simulink model "H8_EMS_partelinealizada"  (R2022b)
settings: Solver=VariableStepAuto  StartTime=0.0  StopTime=10.0  RelTol=1e-3
InitFcn:
  | m = 200;
  | g = 9.81;
  | x_lev12 = 0.443;
  | x_lev34 = 0.542;
  | x_guid12 = 0.4475;
  | x_guid34 = 0.5465;
  | x_lim = 0.0495;
  | y_lev13 = 0.23686;
  | y_lev24 = 0.23686;
  | y_guid13 = 0.24263;
  | y_guid24 = 0.24263;
  | y_lim = 0.0005;
  | y_brk = 0.21552;
  | z_lev = 0.08546;
  | z_guid = 0.026;
  | z_lim = 0.1055;
  | z_brk = 0.03941;
  | kp_lev = 50;
  | ki_lev = 400;
  | kp_guid = 6;
  | ki_guid = 46.5;
  | Imax_lev = 50;
  | Imin_lev = -50;
  | Imax_guid = 50;
  | Imin_guid = 0;
  | cg_nom = 0.567;
  | I = [43.082 0 0; 0 26.887 0; 0 0 29.297]
values from neighbouring files (symbols this model uses):
  cg_suelo = 0.56985    [linealizacion_HEMS.m]
  cg_techo = 0.55735    [linealizacion_HEMS.m]
undefined symbols (not defined in the file or in its folder): ems
libraries: shared6dof x1
settings Model: Creator=USUARIO  LastModifiedBy=USUARIO

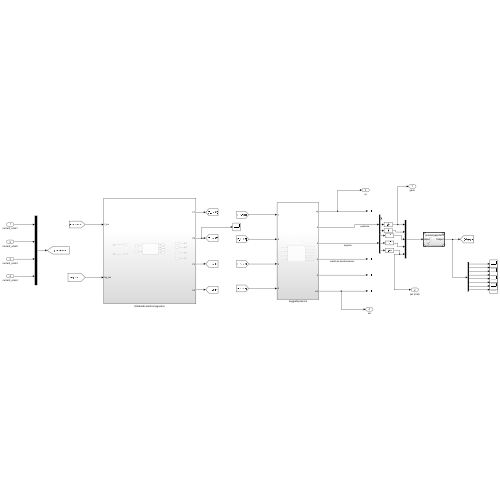
[thumbnail: Simulink's stored preview of the top-level diagram]
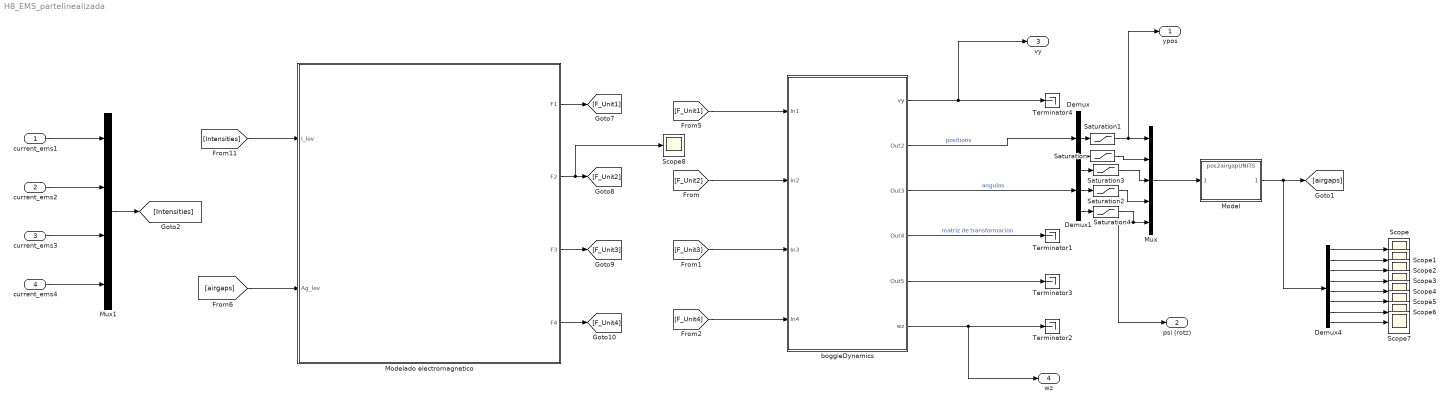
== system H8_EMS_partelinealizada ==
  current_ems1 : Inport
  current_ems2 : Inport  Port=2
  current_ems3 : Inport  Port=3
  current_ems4 : Inport  Port=4
  Demux : Demux  Outputs=3
  Demux1 : Demux  Outputs=3
  Demux4 : Demux  Outputs=8
  Model : ModelReference  ModelNameDialog=pos2airgapUNITS.slx  SimulationMode=Normal  ModelReferenceVersion=1.3
  Modelado electromagnetico : Subsystem
  Mux : Mux  Inputs=5
  Mux1 : Mux
  Saturation : Saturate  UpperLimit=cg_suelo  LowerLimit=cg_techo
  Saturation1 : Saturate  UpperLimit=0.012  LowerLimit=-0.012
  Saturation2 : Saturate  UpperLimit=0.01268  LowerLimit=-0.01268
  Saturation3 : Saturate  UpperLimit=0.0476  LowerLimit=-0.0476
  Saturation4 : Saturate  UpperLimit=0.024  LowerLimit=-0.024
  Scope{,1..8} (9 alike) : Scope
  Terminator{1..4} (4 alike) : Terminator
  boggieDynamics : Subsystem
  ypos : Outport
  psi (rotz) : Outport  Port=2
  vy : Outport  Port=3
  wz : Outport  Port=4
  wires:
  boggieDynamics/3(Out3) -> Demux1/1  "angulos"
  Saturation1/1 -> Mux/1, ypos/1
  boggieDynamics/6(wz) -> wz/1, Terminator2/1
  current_ems3/1 -> Mux1/3
  Demux1/2 -> Saturation2/1
  Demux4/1 -> Scope/1
  boggieDynamics/4(Out4) -> Terminator1/1  "matriz de transformacion"
  Demux4/7 -> Scope6/1
  Saturation/1 -> Mux/2
  current_ems1/1 -> Mux1/1
  [Intensities] -> Modelado electromagnetico/1(I_lev)
  Demux/3 -> Saturation/1
  Demux/2 -> Saturation1/1
  Demux4/4 -> Scope3/1
  Model/1 -> Demux4/1, [airgaps]
  Demux4/3 -> Scope2/1
  Demux4/6 -> Scope5/1
  Saturation4/1 -> psi (rotz)/1, Mux/5
  Mux/1 -> Model/1
  Saturation2/1 -> Mux/4
  Modelado electromagnetico/1(F1) -> [F_Unit1]
  Demux4/8 -> Scope7/1
  [airgaps] -> Modelado electromagnetico/2(Ag_lev)
  Modelado electromagnetico/4(F4) -> [F_Unit4]
  Demux4/2 -> Scope1/1
  Demux4/5 -> Scope4/1
  Demux1/1 -> Saturation3/1
  Demux1/3 -> Saturation4/1
  Saturation3/1 -> Mux/3
  Modelado electromagnetico/3(F3) -> [F_Unit3]
  current_ems4/1 -> Mux1/4
  boggieDynamics/2(Out2) -> Demux/1  "positions"
  Mux1/1 -> [Intensities]
  boggieDynamics/5(Out5) -> Terminator3/1
  boggieDynamics/1(vy) -> vy/1, Terminator4/1
  current_ems2/1 -> Mux1/2
  Modelado electromagnetico/2(F2) -> Scope8/1, [F_Unit2]
  [F_Unit1] -> boggieDynamics/1(In1)
  [F_Unit4] -> boggieDynamics/4(In4)
  [F_Unit3] -> boggieDynamics/3(In3)
  [F_Unit2] -> boggieDynamics/2(In2)

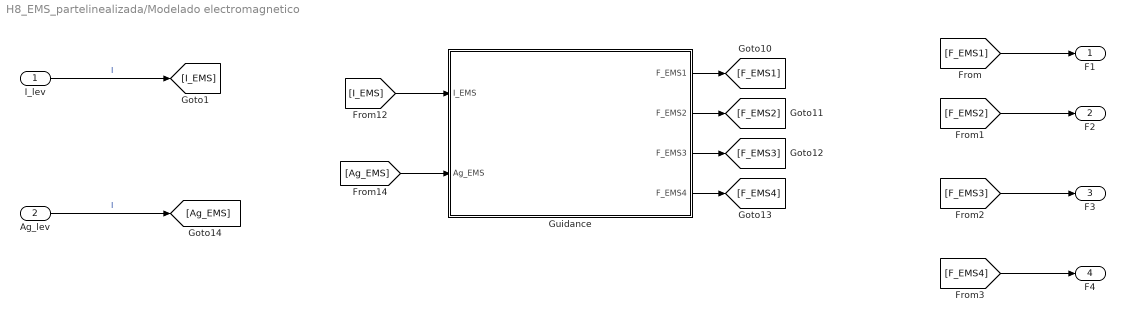
== system H8_EMS_partelinealizada/Modelado electromagnetico ==
  I_lev : Inport
  Ag_lev : Inport  Port=2
  Guidance : Subsystem
  F1 : Outport
  F2 : Outport  Port=2
  F3 : Outport  Port=3
  F4 : Outport  Port=4
  wires:
  I_lev/1 -> [I_EMS]  "I"
  Guidance/2(F_EMS2) -> [F_EMS2]
  Guidance/3(F_EMS3) -> [F_EMS3]
  Guidance/4(F_EMS4) -> [F_EMS4]
  Guidance/1(F_EMS1) -> [F_EMS1]
  [I_EMS] -> Guidance/1(I_EMS)
  [Ag_EMS] -> Guidance/2(Ag_EMS)
  Ag_lev/1 -> [Ag_EMS]  "I"
  [F_EMS2] -> F2/1
  [F_EMS1] -> F1/1
  [F_EMS3] -> F3/1
  [F_EMS4] -> F4/1

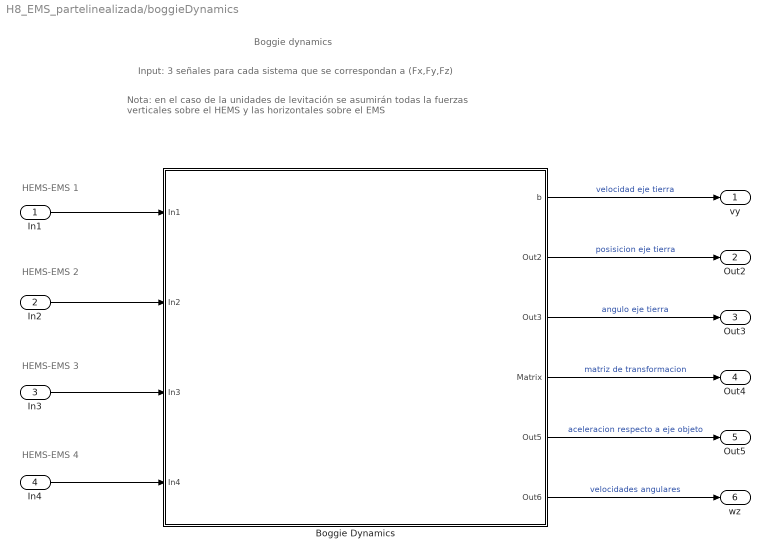
== system H8_EMS_partelinealizada/boggieDynamics ==
  note: Input: 3 señales para cada sistema que se correspondan a (Fx,Fy,Fz)
  note: HEMS-EMS 3
  note: HEMS-EMS 1
  note: HEMS-EMS 4
  note: HEMS-EMS 2
  note: Boggie dynamics
  note: Nota: en el caso de la unidades de levitación se asumirán todas la fuerzas
      | verticales sobre el HEMS y las horizontales sobre el EMS
  In1 : Inport
  In2 : Inport  Port=2
  In3 : Inport  Port=3
  In4 : Inport  Port=4
  Boggie Dynamics : Subsystem
      mask Display: image('C:\UPV\Hyperloop\Levitacion\ejes.png'); % Use "Edit Image" on toolstrip to change.
  vy : Outport
  Out2 : Outport  Port=2
  Out3 : Outport  Port=3
  Out4 : Outport  Port=4
  Out5 : Outport  Port=5
  wz : Outport  Port=6
  wires:
  Boggie Dynamics/4(Matrix) -> Out4/1  "matriz de transformacion"
  Boggie Dynamics/6(Out6) -> wz/1  "velocidades angulares"
  Boggie Dynamics/5(Out5) -> Out5/1  "aceleracion respecto a eje objeto"
  In1/1 -> Boggie Dynamics/1(In1)
  In3/1 -> Boggie Dynamics/3(In3)
  In4/1 -> Boggie Dynamics/4(In4)
  Boggie Dynamics/1(b) -> vy/1  "velocidad eje tierra"
  In2/1 -> Boggie Dynamics/2(In2)
  Boggie Dynamics/2(Out2) -> Out2/1  "posisicion eje tierra"
  Boggie Dynamics/3(Out3) -> Out3/1  "angulo eje tierra"

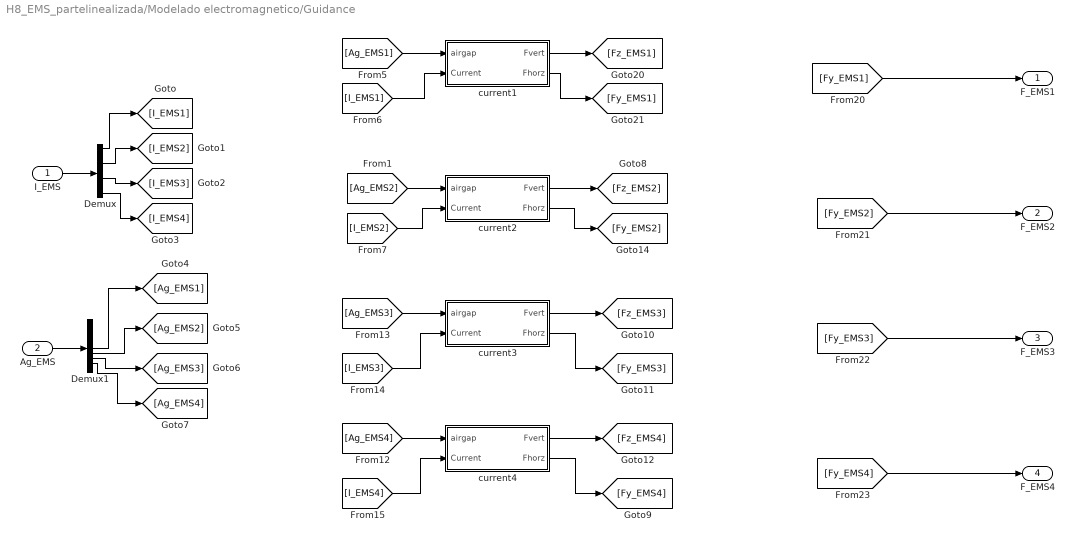
== system H8_EMS_partelinealizada/Modelado electromagnetico/Guidance ==
  I_EMS : Inport
  Ag_EMS : Inport  Port=2
  Demux : Demux
  Demux1 : Demux  Outputs=8
  current1 : Subsystem
  current2 : Subsystem
  current3 : Subsystem
  current4 : Subsystem
  F_EMS1 : Outport
  F_EMS2 : Outport  Port=2
  F_EMS3 : Outport  Port=3
  F_EMS4 : Outport  Port=4
  wires:
  I_EMS/1 -> Demux/1
  [Fy_EMS2] -> F_EMS2/1
  Demux/2 -> [I_EMS2]
  [Fy_EMS4] -> F_EMS4/1
  [Fy_EMS1] -> F_EMS1/1
  [Fy_EMS3] -> F_EMS3/1
  Ag_EMS/1 -> Demux1/1
  Demux/1 -> [I_EMS1]
  Demux/4 -> [I_EMS4]
  Demux/3 -> [I_EMS3]
  current1/1(Fvert) -> [Fz_EMS1]
  current1/2(Fhorz) -> [Fy_EMS1]
  [Ag_EMS1] -> current1/1(airgap)
  [I_EMS1] -> current1/2(Current)
  current2/1(Fvert) -> [Fz_EMS2]
  [Ag_EMS2] -> current2/1(airgap)
  [I_EMS2] -> current2/2(Current)
  current2/2(Fhorz) -> [Fy_EMS2]
  current3/1(Fvert) -> [Fz_EMS3]
  [Ag_EMS3] -> current3/1(airgap)
  current4/1(Fvert) -> [Fz_EMS4]
  [I_EMS3] -> current3/2(Current)
  current4/2(Fhorz) -> [Fy_EMS4]
  current3/2(Fhorz) -> [Fy_EMS3]
  [Ag_EMS4] -> current4/1(airgap)
  [I_EMS4] -> current4/2(Current)
  Demux1/8 -> [Ag_EMS4]
  Demux1/7 -> [Ag_EMS3]
  Demux1/6 -> [Ag_EMS2]
  Demux1/5 -> [Ag_EMS1]

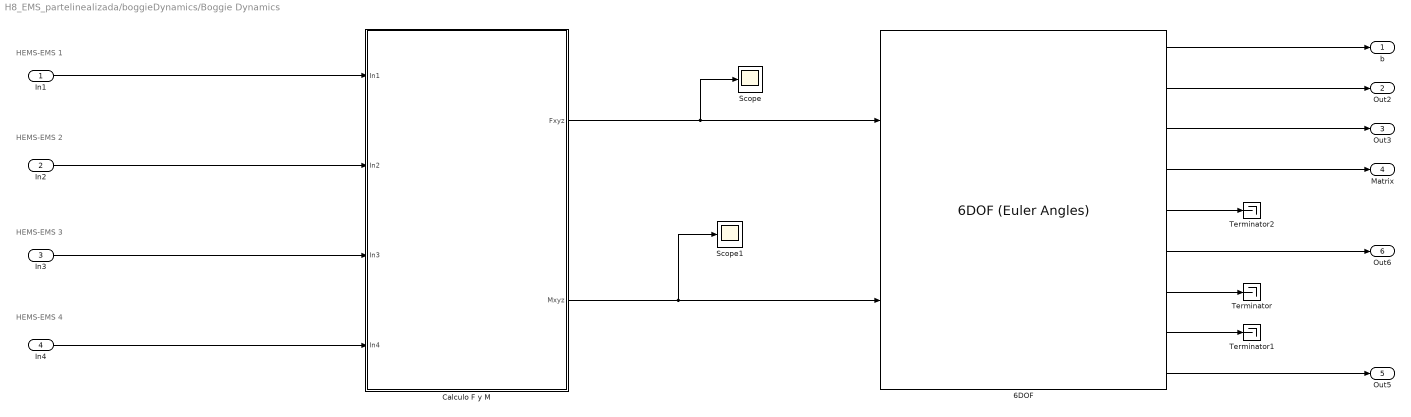
== system H8_EMS_partelinealizada/boggieDynamics/Boggie Dynamics ==
  note: HEMS-EMS 1
  note: HEMS-EMS 2
  note: HEMS-EMS 3
  note: HEMS-EMS 4
  In1 : Inport
  In2 : Inport  Port=2
  In3 : Inport  Port=3
  In4 : Inport  Port=4
  "6DOF " : shared6dof/6DOF (Euler Angles)  units=Metric (MKS)  mtype=Fixed  rep=Euler Angles  xme_0=[0 0.00 cg_nom]  Vm_0=[0 0 0]  eul_0=[0 0 0.00]  pm_0=[0 0 0]  mass_0=m  mass_e=0.5  mass_f=2.0  inertia=I  inertia_e=eye(3)  inertia_f=2*eye(3)  k_quat=1.0  vre_flag=on  abi_flag=on  aMode=0  xme_statename=''  Vm_statename=''  eul_statename=''  quat_statename=''  pm_statename=''  mass_statename=''
  Calculo F y M : Subsystem
  Scope : Scope
  Scope1 : Scope
  Terminator : Terminator
  Terminator1 : Terminator
  Terminator2 : Terminator
  b : Outport
  Out2 : Outport  Port=2
  Out3 : Outport  Port=3
  Matrix : Outport  Port=4
  Out5 : Outport  Port=5
  Out6 : Outport  Port=6
  wires:
  "6DOF "/1 -> b/1
  "6DOF "/2 -> Out2/1
  "6DOF "/3 -> Out3/1
  In1/1 -> Calculo F y M/1(In1)
  In2/1 -> Calculo F y M/2(In2)
  In3/1 -> Calculo F y M/3(In3)
  In4/1 -> Calculo F y M/4(In4)
  "6DOF "/6 -> Out6/1
  "6DOF "/8 -> Terminator1/1
  "6DOF "/7 -> Terminator/1
  Calculo F y M/1(Fxyz) -> Scope/1, "6DOF "/1
  Calculo F y M/2(Mxyz) -> Scope1/1, "6DOF "/2
  "6DOF "/4 -> Matrix/1
  "6DOF "/9 -> Out5/1
  "6DOF "/5 -> Terminator2/1

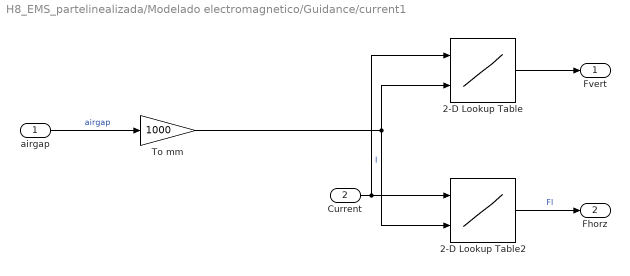
== system H8_EMS_partelinealizada/Modelado electromagnetico/Guidance/current1 ==
  airgap : Inport
  Current : Inport  Port=2
  2-D Lookup Table : Lookup_n-D  BreakpointsForDimension1=ems.Current  BreakpointsForDimension2=ems.Airgap'  Table=ems.Force_Vertical  InternalRulePriority=Speed  RndMeth=Simplest
      settings: InputPortMap=u0,u1
  2-D Lookup Table2 : Lookup_n-D  BreakpointsForDimension1=ems.Current  BreakpointsForDimension2=ems.Airgap'  Table=ems.Force_Horizontal  InternalRulePriority=Speed  RndMeth=Simplest
      settings: InputPortMap=u0,u1
  To mm : Gain  Gain=1000
  Fvert : Outport
  Fhorz : Outport  Port=2
  wires:
  2-D Lookup Table2/1 -> Fhorz/1  "Fl"
  Current/1 -> 2-D Lookup Table2/1, 2-D Lookup Table/1  "I"
  2-D Lookup Table/1 -> Fvert/1
  airgap/1 -> To mm/1  "airgap"
  To mm/1 -> 2-D Lookup Table/2, 2-D Lookup Table2/2

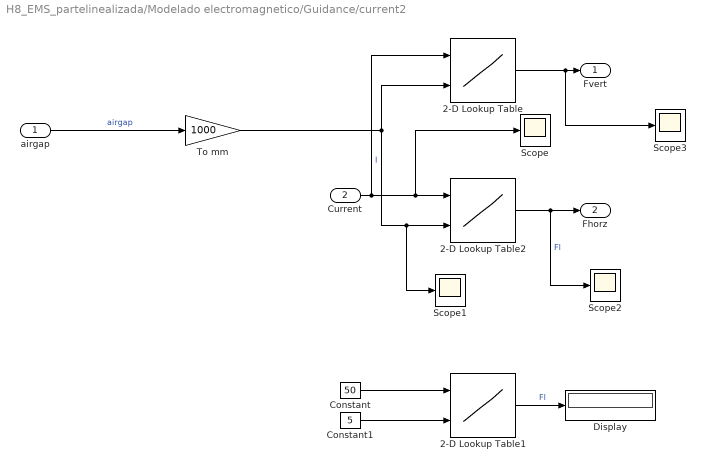
== system H8_EMS_partelinealizada/Modelado electromagnetico/Guidance/current2 ==
  airgap : Inport
  Current : Inport  Port=2
  2-D Lookup Table : Lookup_n-D  BreakpointsForDimension1=ems.Current  BreakpointsForDimension2=ems.Airgap'  Table=ems.Force_Vertical  InternalRulePriority=Speed  RndMeth=Simplest
      settings: InputPortMap=u0,u1
  2-D Lookup Table1 : Lookup_n-D  BreakpointsForDimension1=ems.Current  BreakpointsForDimension2=ems.Airgap'  Table=ems.Force_Horizontal  InternalRulePriority=Speed  RndMeth=Simplest
      settings: InputPortMap=u0,u1
  2-D Lookup Table2 : Lookup_n-D  BreakpointsForDimension1=ems.Current  BreakpointsForDimension2=ems.Airgap'  Table=ems.Force_Horizontal  InternalRulePriority=Speed  RndMeth=Simplest
      settings: InputPortMap=u0,u1
  Constant : Constant  Value=50
  Constant1 : Constant  Value=5
  Display : Display
  Scope{,1..3} (4 alike) : Scope
  To mm : Gain  Gain=1000
  Fvert : Outport
  Fhorz : Outport  Port=2
  wires:
  2-D Lookup Table2/1 -> Scope2/1, Fhorz/1  "Fl"
  Current/1 -> Scope/1, 2-D Lookup Table2/1, 2-D Lookup Table/1  "I"
  airgap/1 -> To mm/1  "airgap"
  To mm/1 -> Scope1/1, 2-D Lookup Table2/2, 2-D Lookup Table/2
  2-D Lookup Table/1 -> Scope3/1, Fvert/1
  Constant/1 -> 2-D Lookup Table1/1
  Constant1/1 -> 2-D Lookup Table1/2
  2-D Lookup Table1/1 -> Display/1  "Fl"

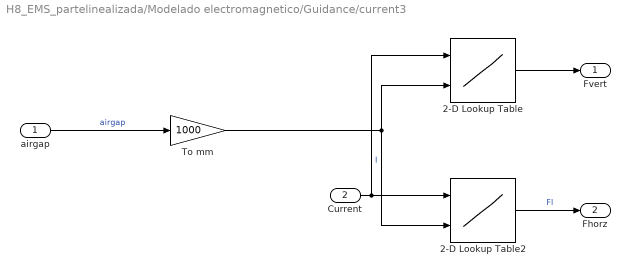
== system H8_EMS_partelinealizada/Modelado electromagnetico/Guidance/current3 ==
  airgap : Inport
  Current : Inport  Port=2
  2-D Lookup Table : Lookup_n-D  BreakpointsForDimension1=ems.Current  BreakpointsForDimension2=ems.Airgap'  Table=ems.Force_Vertical  InternalRulePriority=Speed  RndMeth=Simplest
      settings: InputPortMap=u0,u1
  2-D Lookup Table2 : Lookup_n-D  BreakpointsForDimension1=ems.Current  BreakpointsForDimension2=ems.Airgap'  Table=ems.Force_Horizontal  InternalRulePriority=Speed  RndMeth=Simplest
      settings: InputPortMap=u0,u1
  To mm : Gain  Gain=1000
  Fvert : Outport
  Fhorz : Outport  Port=2
  wires:
  2-D Lookup Table2/1 -> Fhorz/1  "Fl"
  Current/1 -> 2-D Lookup Table2/1, 2-D Lookup Table/1  "I"
  2-D Lookup Table/1 -> Fvert/1
  airgap/1 -> To mm/1  "airgap"
  To mm/1 -> 2-D Lookup Table/2, 2-D Lookup Table2/2

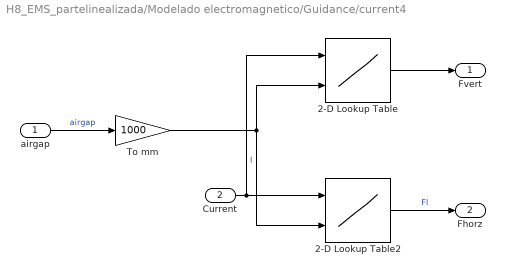
== system H8_EMS_partelinealizada/Modelado electromagnetico/Guidance/current4 ==
  airgap : Inport
  Current : Inport  Port=2
  2-D Lookup Table : Lookup_n-D  BreakpointsForDimension1=ems.Current  BreakpointsForDimension2=ems.Airgap'  Table=ems.Force_Vertical  InternalRulePriority=Speed  RndMeth=Simplest
      settings: InputPortMap=u0,u1
  2-D Lookup Table2 : Lookup_n-D  BreakpointsForDimension1=ems.Current  BreakpointsForDimension2=ems.Airgap'  Table=ems.Force_Horizontal  InternalRulePriority=Speed  RndMeth=Simplest
      settings: InputPortMap=u0,u1
  To mm : Gain  Gain=1000
  Fvert : Outport
  Fhorz : Outport  Port=2
  wires:
  2-D Lookup Table2/1 -> Fhorz/1  "Fl"
  Current/1 -> 2-D Lookup Table2/1, 2-D Lookup Table/1  "I"
  2-D Lookup Table/1 -> Fvert/1
  airgap/1 -> To mm/1  "airgap"
  To mm/1 -> 2-D Lookup Table/2, 2-D Lookup Table2/2

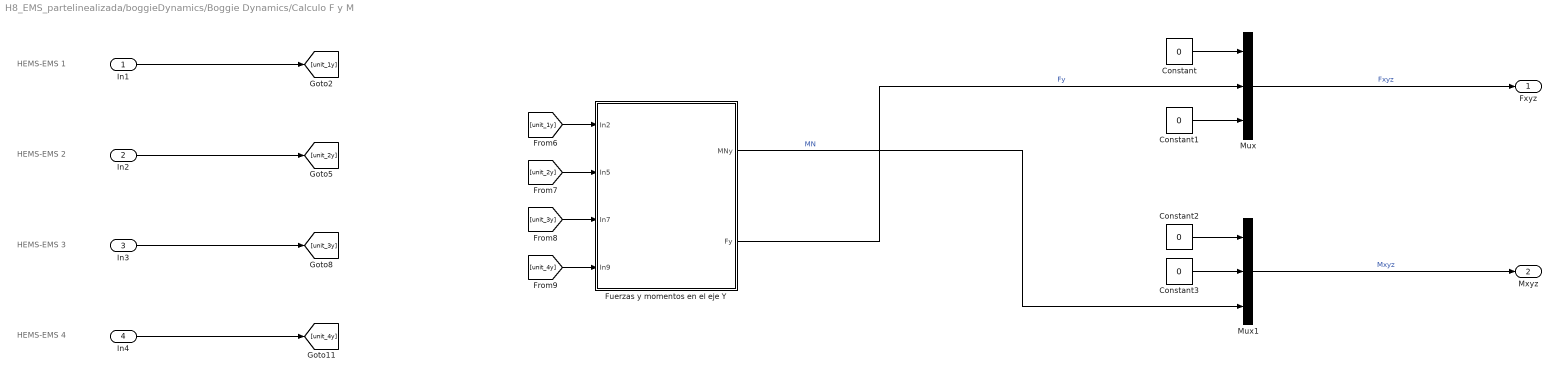
== system H8_EMS_partelinealizada/boggieDynamics/Boggie Dynamics/Calculo F y M ==
  note: HEMS-EMS 3
  note: HEMS-EMS 1
  note: HEMS-EMS 4
  note: HEMS-EMS 2
  In1 : Inport
  In2 : Inport  Port=2
  In3 : Inport  Port=3
  In4 : Inport  Port=4
  Constant{,1..3} (4 alike) : Constant  Value=0
  Fuerzas y momentos en el eje Y : Subsystem
  Mux : Mux  Inputs=3
  Mux1 : Mux  Inputs=3
  Fxyz : Outport
  Mxyz : Outport  Port=2
  wires:
  Mux/1 -> Fxyz/1  "Fxyz"
  Mux1/1 -> Mxyz/1  "Mxyz"
  Fuerzas y momentos en el eje Y/1(MNy) -> Mux1/3  "MN"
  Fuerzas y momentos en el eje Y/2(Fy) -> Mux/2  "Fy"
  In4/1 -> [unit_4y]
  In3/1 -> [unit_3y]
  In2/1 -> [unit_2y]
  In1/1 -> [unit_1y]
  [unit_4y] -> Fuerzas y momentos en el eje Y/4(In9)
  [unit_1y] -> Fuerzas y momentos en el eje Y/1(In2)
  [unit_2y] -> Fuerzas y momentos en el eje Y/2(In5)
  [unit_3y] -> Fuerzas y momentos en el eje Y/3(In7)
  Constant/1 -> Mux/1
  Constant1/1 -> Mux/3
  Constant2/1 -> Mux1/1
  Constant3/1 -> Mux1/2

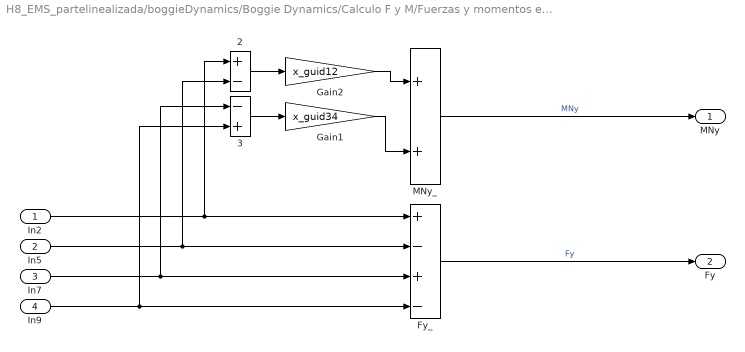
== system H8_EMS_partelinealizada/boggieDynamics/Boggie Dynamics/Calculo F y M/Fuerzas y momentos en el eje Y ==
  In2 : Inport
  In5 : Inport  Port=2
  In7 : Inport  Port=3
  In9 : Inport  Port=4
  " 2" : Sum  Inputs=+-
  " 3" : Sum  Inputs=-+
  Fy_ : Sum  Inputs=+-+-
  Gain1 : Gain  Gain=x_guid34
  Gain2 : Gain  Gain=x_guid12
  MNy_ : Sum
  MNy : Outport
  Fy : Outport  Port=2
  wires:
  Fy_/1 -> Fy/1  "Fy"
  In7/1 -> " 3"/1, Fy_/3
  In9/1 -> " 3"/2, Fy_/4
  In2/1 -> " 2"/1, Fy_/1
  In5/1 -> " 2"/2, Fy_/2
  MNy_/1 -> MNy/1  "MNy"
  " 3"/1 -> Gain1/1
  " 2"/1 -> Gain2/1
  Gain1/1 -> MNy_/2
  Gain2/1 -> MNy_/1
